simulink model "clik_inverse"  (R2022b)
settings: Solver=VariableStepAuto  StartTime=0.0  StopTime=4  FixedStep=0.001  RelTol=1e-3
undefined symbols (not defined in the file or in its folder): DiscIntNeverNeededParam, q0, Tc
settings Model: Creator=Xp  LastModifiedBy=DELL
settings SolverCC: AlgebraicLoopSolver=TrustRegion
settings DataIOCC: LimitDataPoints=on  SaveFormat=Array  SignalLoggingSaveFormat=ModelDataLogs  ReturnWorkspaceOutputs=off
settings OptimizationCC: ExpressionDepthLimit=2147483647  InitFltsAndDblsToZero=on  LifeSpan=inf
settings DebuggingCC: SaveWithParameterizedLinksMsg=none  UnderspecifiedInitializationDetection=Classic  MergeDetectMultiDrivingBlocksExec=none  SolverPrmCheckMsg=warning  MultiTaskDSMMsg=warning  MultiTaskCondExecSysMsg=none  FcnCallInpInsideContextMsg=warning  UnconnectedInputMsg=warning  UnconnectedOutputMsg=warning  UnconnectedLineMsg=warning  StateNameClashWarn=warning  SFUnexpectedBacktrackingDiag=warning  SFNoUnconditionalDefaultTransitionDiag=warning  SFExecutionAtInitializationDiag=none  SFMachineParentedDataDiag=warning  ArithmeticOperatorsInVariantConditions=warning
settings HardwareCC: ProdBitPerPointer=32  ProdBitPerSizeT=32  ProdBitPerPtrDiffT=32  ProdLargestAtomicFloat=None  ProdIntDivRoundTo=Undefined  ProdEndianess=Unspecified  ProdWordSize=32  ProdHWDeviceType=32-bit Generic
settings ModelReferenceCC: EnableRefExpFcnMdlSchedulingChecks=on  PropagateSignalLabelsOutOfModel=off
settings SFSimCC: CustomCodeUndefinedFunction=UseInterfaceOnly
settings RTWCC: DLArmComputeVersion=19.05
settings CodeAppCC: StateflowObjectComments=on
settings GRTTargetCC: TargetLangStandard=C89/C90 (ANSI)  CombineOutputUpdateFcns=off  GRTInterface=on
settings ConfigComp: CovMetricSettings=dw  CovSaveCumulativeToWorkspaceVar=on  CovSaveSingleToWorkspaceVar=on

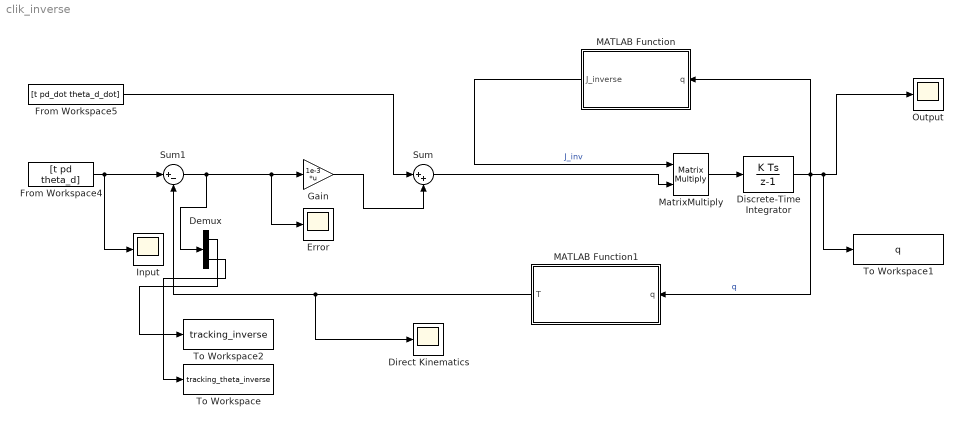
== system clik_inverse ==
  Demux : Demux  Outputs=2
  Direct Kinematics : Scope
  Discrete-Time Integrator : DiscreteIntegrator  InitialCondition=q0  SampleTime=Tc  LimitOutput=on  UpperSaturationLimit=[pi/2;pi/4;1;2*pi]  LowerSaturationLimit=[-pi/2;-pi/2;0.25;-2*pi]  ICPrevOutput=DiscIntNeverNeededParam  ICPrevScaledInput=DiscIntNeverNeededParam
  Error : Scope
  From Workspace4 : FromWorkspace  VariableName=[t pd theta_d]  SampleTime=Tc
  From Workspace5 : FromWorkspace  VariableName=[t pd_dot theta_d_dot]  SampleTime=Tc
  Gain : Gain  Gain=1e-3  Multiplication=Matrix(K*u)
  Input : Scope
  MATLAB Function : MATLAB Function  TreatAsAtomicUnit=on
  MATLAB Function1 : MATLAB Function  TreatAsAtomicUnit=on
  MatrixMultiply : Product  Multiplication=Matrix(*)
  Output : Scope
  Sum : Sum  Inputs=|++
  Sum1 : Sum  Inputs=|+-
  To Workspace : ToWorkspace  VariableName=tracking_theta_inverse  SampleTime=Tc
  To Workspace1 : ToWorkspace  VariableName=q  SampleTime=Tc
      settings: Save2DSignal=2-D array (concatenate along first dimension)
  To Workspace2 : ToWorkspace  VariableName=tracking_inverse  SampleTime=Tc
  wires:
  Discrete-Time Integrator/1 -> MATLAB Function/1(q), To Workspace1/1, Output/1, MATLAB Function1/1(q)  "q"
  From Workspace5/1 -> Sum/1
  MATLAB Function/1(J_inverse) -> MatrixMultiply/1  "J_inv"
  Sum/1 -> MatrixMultiply/2
  MatrixMultiply/1 -> Discrete-Time Integrator/1
  Sum1/1 -> Demux/1, Error/1, Gain/1
  Gain/1 -> Sum/2
  From Workspace4/1 -> Sum1/1, Input/1
  MATLAB Function1/1(T) -> Direct Kinematics/1, Sum1/2
  Demux/1 -> To Workspace2/1
  Demux/2 -> To Workspace/1

== matlab function clik_inverse/MATLAB Function1 ==
  data: q input; T output
function T = direct_kin(q)

% Defining link length values
a1 = 0.5;
a2 = 0.5;
d0 = 1;

% Assigning individual joint values to the corresponding rows of the
% q(angle) being taken as input
q1=q(1);
q2=q(2);
d3=q(3);
q4=q(4);

% Obtained Rotation and translation direct kinematics matrix for scara manipulator
R=[cos(q1+q2+q4),sin(q1+q2+q4),0;sin(q1+q2+q4),-cos(q1+q2+q4),0;0,0,-1;0 0 0];
T=[a1*cos(q1)+a2*cos(q1+q2);a1*sin(q1)+a2*sin(q1+q2);-d3+d0;q1+q2+q4];

== matlab function clik_inverse/MATLAB Function ==
  data: q input; J_inverse output
function J_inverse = jacobian_inverse(q)

% Calling the jacobian function from the jacobian matlab file
J = jacobian(q);

% Calculating inverse of jacobian matrix
J_inverse = inv(J);
